simulink model "BLAC0_coppia"  (R2025b)
settings: Solver=FixedStepAuto  StartTime=0.0  StopTime=0.2  FixedStep=1e-5  RelTol=1e-3
values from neighbouring files (symbols this model uses):
  B = 3.8e-005    (= 3.8e-05)    [Dati0_1.m]
  J = 0.0000251    (= 2.51e-05)    [Dati0_1.m]
  Kc = ms*np*lambdaf/2    (= 0.27)    [Dati0_1.m]
  Lsd = 0.005/2    (= 0.0025)    [Dati0_1.m]
  Lsq = Lsd    (= 0.0025)    [Dati0_1.m]
  np = 2    [Dati0_1.m]
  PSIPM = lambdaf    (= 0.09)    [Dati0_1.m]
  Rs = 3.1/2    (= 1.55)    [Dati0_1.m]
  wrr = 1256.6    [Dati0_1.m]
settings Model: Creator=rosco  LastModifiedBy=Steph

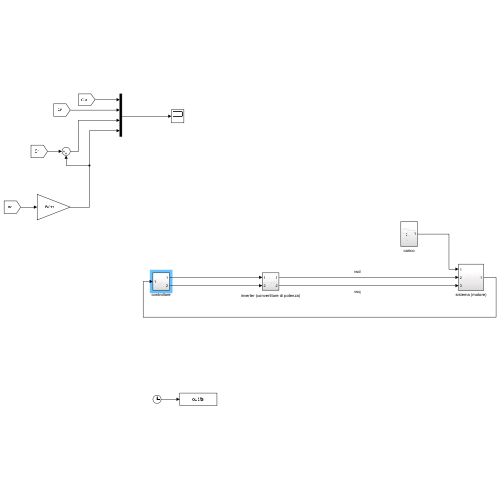
[thumbnail: Simulink's stored preview of the top-level diagram]
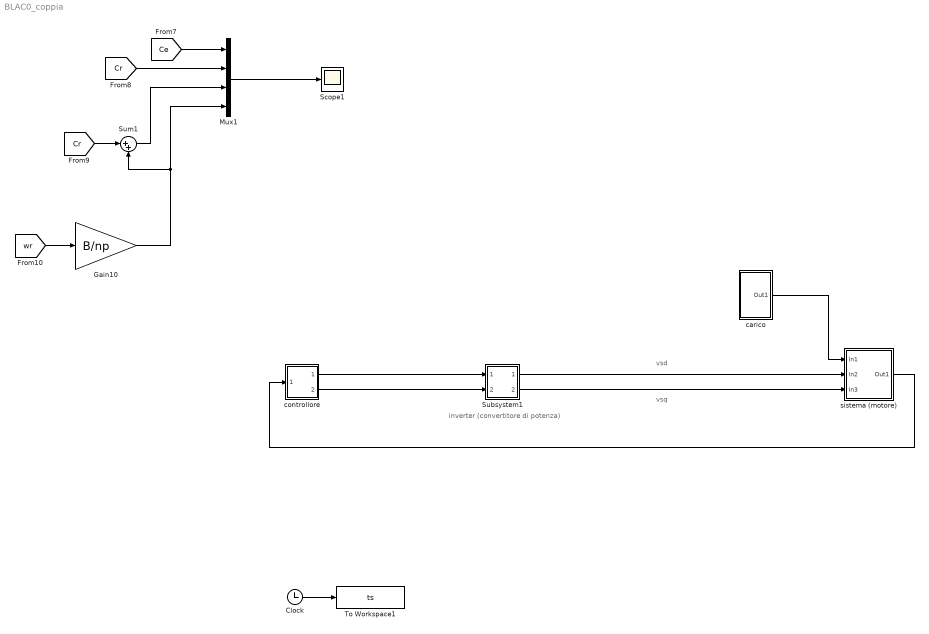
== system BLAC0_coppia ==
  note: vsq
  note: vsd
  note: inverter (convertitore di potenza)
  Clock : Clock
  Gain10 : Gain  Gain=B/np
  Mux1 : Mux
  Scope1 : Scope
      settings: ActiveDisplayYMinimum=-0.074999999999999026  ActiveDisplayYMaximum=0.67499999999999138  DataLoggingVariableName=ScopeData2
  Subsystem1 : Subsystem
  Sum1 : Sum  Inputs=|++
  To Workspace1 : ToWorkspace  VariableName=ts  SaveFormat=Timeseries  SampleTime=-1
  carico : Subsystem
  controllore : Subsystem
  sistema (motore) : Subsystem
  wires:
  Clock/1 -> To Workspace1/1
  [Cr] -> Sum1/1
  [wr] -> Gain10/1
  Gain10/1 -> Sum1/2, Mux1/4
  Sum1/1 -> Mux1/3
  [Cr] -> Mux1/2
  [Ce] -> Mux1/1
  Mux1/1 -> Scope1/1
  controllore/1(Out1) -> Subsystem1/1(In1)
  controllore/2(Out2) -> Subsystem1/2(In2)
  carico/1(Out1) -> sistema (motore)/1(In1)
  Subsystem1/1(Out1) -> sistema (motore)/2(In2)
  Subsystem1/2(Out2) -> sistema (motore)/3(In3)
  sistema (motore)/1(Out1) -> controllore/1(In1)

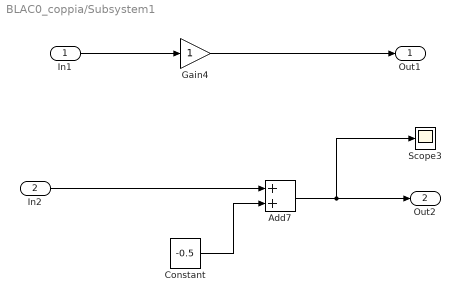
== system BLAC0_coppia/Subsystem1 ==
  In1 : Inport
  In2 : Inport  Port=2
  Add7 : Sum
  Constant : Constant  Value=-0.5
  Gain4 : Gain
  Scope3 : Scope
      settings: ActiveDisplayYMinimum=-10.413828677585377  ActiveDisplayYMaximum=128.16890254271289
  Out1 : Outport
  Out2 : Outport  Port=2
  wires:
  In2/1 -> Add7/1
  In1/1 -> Gain4/1
  Constant/1 -> Add7/2
  Add7/1 -> Out2/1, Scope3/1
  Gain4/1 -> Out1/1

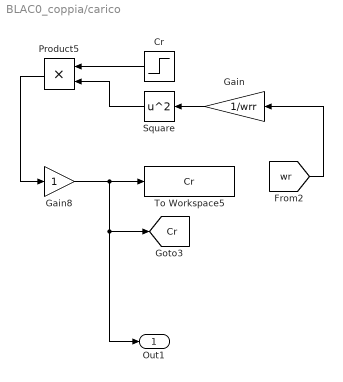
== system BLAC0_coppia/carico ==
  Cr : Step  Time=0  After=0.6  SampleTime=0
  Gain : Gain  Gain=1/wrr
  Gain8 : Gain
  Product5 : Product
  Square : Math  Operator=square
  To Workspace5 : ToWorkspace  VariableName=Cr  SaveFormat=Timeseries  SampleTime=-1
  Out1 : Outport
  tag scope: Cr=global
  wires:
  Gain/1 -> Square/1
  [wr] -> Gain/1
  Gain8/1 -> To Workspace5/1, Out1/1, [Cr]
  Cr/1 -> Product5/1
  Product5/1 -> Gain8/1
  Square/1 -> Product5/2

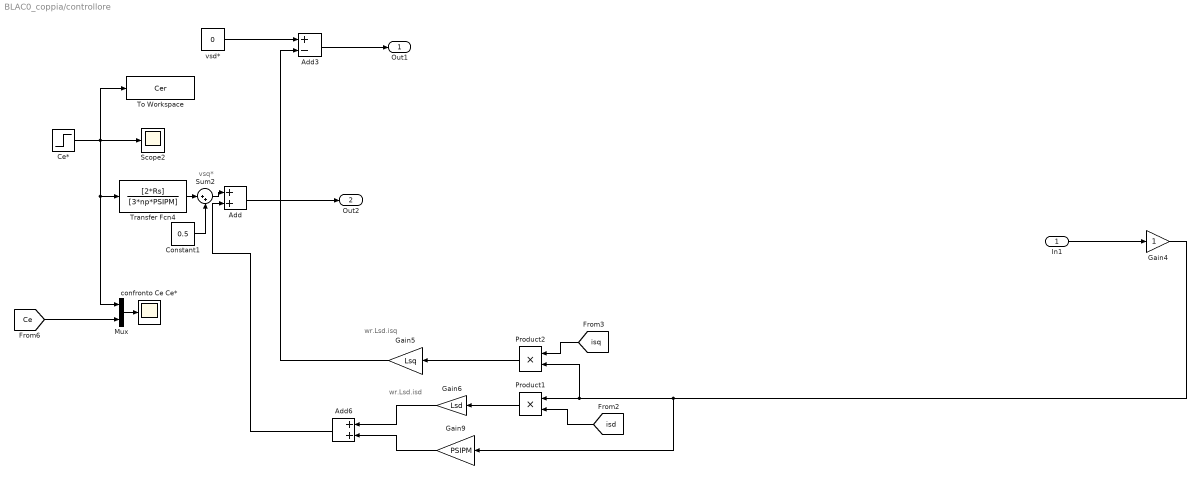
== system BLAC0_coppia/controllore ==
  note: vsq*
  note: wr.Lsd.isq
  note: wr.Lsd.isd
  In1 : Inport
  Add : Sum
  Add3 : Sum  Inputs=+-
  Add6 : Sum
  Ce* : Step  Time=0  After=0.6  SampleTime=0
  Constant1 : Constant  Value=0.5
  Gain4 : Gain
  Gain5 : Gain  Gain=Lsq
  Gain6 : Gain  Gain=Lsd
  Gain9 : Gain  Gain=PSIPM
  Mux : Mux  Inputs=2
  Product1 : Product
  Product2 : Product
  Scope2 : Scope
      settings: ActiveDisplayYMinimum=-1  ActiveDisplayYMaximum=1  DataLoggingVariableName=ScopeData2
  Sum2 : Sum  Inputs=|++
  To Workspace : ToWorkspace  VariableName=Cer  SaveFormat=Timeseries  SampleTime=-1
  Transfer Fcn4 : TransferFcn  Numerator=[2*Rs]  Denominator=[3*np*PSIPM]
  confronto Ce Ce* : Scope
      settings: ActiveDisplayYMinimum=0.29519  ActiveDisplayYMaximum=0.61079
  vsd* : Constant  Value=0
  Out1 : Outport
  Out2 : Outport  Port=2
  wires:
  [isd] -> Product1/2
  Gain6/1 -> Add6/1
  Gain5/1 -> Add3/2
  Ce*/1 -> Mux/1, Transfer Fcn4/1, To Workspace/1, Scope2/1
  Gain4/1 -> Gain9/1, Product2/2, Product1/1
  [isq] -> Product2/1
  Mux/1 -> confronto Ce Ce*/1
  [Ce] -> Mux/2
  Transfer Fcn4/1 -> Sum2/1
  Product2/1 -> Gain5/1
  Product1/1 -> Gain6/1
  Add6/1 -> Add/2
  Gain9/1 -> Add6/2
  Sum2/1 -> Add/1
  vsd*/1 -> Add3/1
  Add3/1 -> Out1/1
  In1/1 -> Gain4/1
  Add/1 -> Out2/1
  Constant1/1 -> Sum2/2

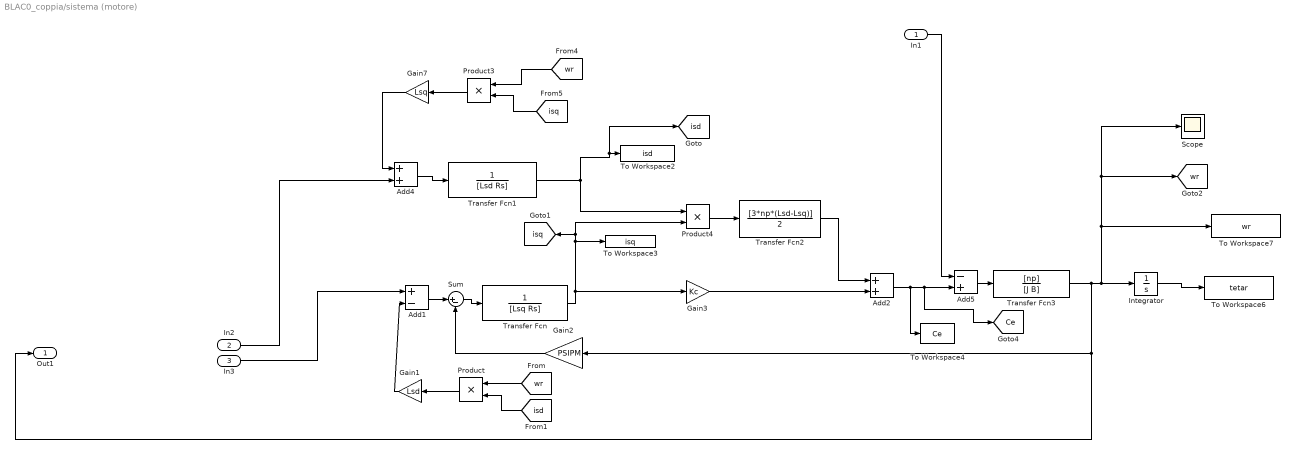
== system BLAC0_coppia/sistema (motore) ==
  In1 : Inport
  In2 : Inport  Port=2
  In3 : Inport  Port=3
  Add1 : Sum  Inputs=+-
  Add2 : Sum
  Add4 : Sum
  Add5 : Sum  Inputs=-+
  Gain1 : Gain  Gain=Lsd
  Gain2 : Gain  Gain=PSIPM
  Gain3 : Gain  Gain=Kc
  Gain7 : Gain  Gain=Lsq
  Integrator : Integrator
  Product : Product
  Product3 : Product
  Product4 : Product
  Scope : Scope
      settings: ActiveDisplayYMinimum=-153.98081246699803  ActiveDisplayYMaximum=1385.8273122029825
  Sum : Sum  Inputs=|+-
  To Workspace2 : ToWorkspace  VariableName=isd  SaveFormat=Timeseries  SampleTime=-1
  To Workspace3 : ToWorkspace  VariableName=isq  SaveFormat=Timeseries  SampleTime=-1
  To Workspace4 : ToWorkspace  VariableName=Ce  SaveFormat=Timeseries  SampleTime=-1
  To Workspace6 : ToWorkspace  VariableName=tetar  SaveFormat=Timeseries  SampleTime=-1
  To Workspace7 : ToWorkspace  VariableName=wr  SaveFormat=Timeseries  SampleTime=-1
  Transfer Fcn : TransferFcn  Denominator=[Lsq Rs]
  Transfer Fcn1 : TransferFcn  Denominator=[Lsd Rs]
  Transfer Fcn2 : TransferFcn  Numerator=[3*np*(Lsd-Lsq)]  Denominator=[2]
  Transfer Fcn3 : TransferFcn  Numerator=[np]  Denominator=[J B]
  Out1 : Outport
  tag scope: Ce=global, isd=global, isq=global, wr=global
  wires:
  Add2/1 -> To Workspace4/1, [Ce], Add5/2
  Sum/1 -> Transfer Fcn/1
  Transfer Fcn/1 -> To Workspace3/1, [isq], Product4/2, Gain3/1
  Transfer Fcn2/1 -> Add2/1
  In3/1 -> Add1/1
  [isq] -> Product3/2
  Gain1/1 -> Add1/2
  Gain7/1 -> Add4/1
  [wr] -> Product3/1
  [wr] -> Product/1
  Add1/1 -> Sum/1
  Gain2/1 -> Sum/2
  Gain3/1 -> Add2/2
  Add5/1 -> Transfer Fcn3/1
  Transfer Fcn1/1 -> [isd], To Workspace2/1, Product4/1
  Product3/1 -> Gain7/1
  Add4/1 -> Transfer Fcn1/1
  Transfer Fcn3/1 -> Out1/1, Gain2/1, To Workspace7/1, Scope/1, [wr], Integrator/1
  Product4/1 -> Transfer Fcn2/1
  [isd] -> Product/2
  Integrator/1 -> To Workspace6/1
  Product/1 -> Gain1/1
  In1/1 -> Add5/1
  In2/1 -> Add4/2
